simulink model "untitled"  (R2023b)
settings: Solver=VariableStepAuto  StartTime=0.0  StopTime=10.0  RelTol=1e-3
settings Model: Creator=ray  LastModifiedBy=ray

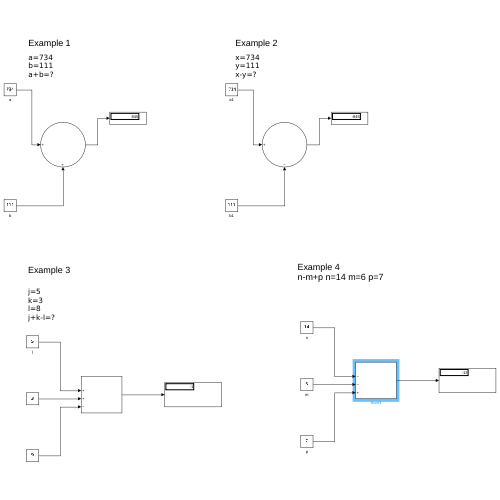
[thumbnail: Simulink's stored preview of the top-level diagram]
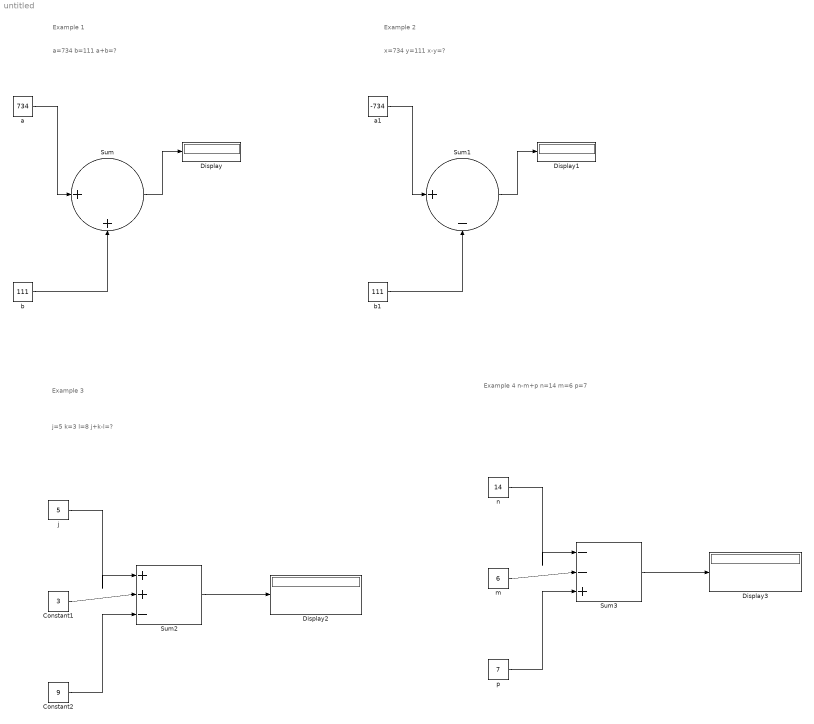
== system untitled ==
  note: a=734
      | b=111
      | a+b=?
  note: Example 1
  note: x=734
      | y=111
      | x-y=?
  note: Example 2
  note: Example 3
  note: j=5
      | k=3
      | l=8
      | j+k-l=?
  note: Example 4
      | n-m+p n=14 m=6 p=7
  Constant1 : Constant  Value=3
  Constant2 : Constant  Value=9
  Display{,1..3} (4 alike) : Display
  Sum : Sum  Inputs=|++
  Sum1 : Sum  Inputs=|+-
  Sum2 : Sum  Inputs=|++-
  Sum3 : Sum  Inputs=|--+
  a : Constant  Value=734
  a1 : Constant  Value=-734
  b : Constant  Value=111
  b1 : Constant  Value=111
  j : Constant  Value=5
  m : Constant  Value=6
  n : Constant  Value=14
  p : Constant  Value=7
  wires:
  a/1 -> Sum/1
  b/1 -> Sum/2
  Sum/1 -> Display/1
  a1/1 -> Sum1/1
  Sum1/1 -> Display1/1
  b1/1 -> Sum1/2
  j/1 -> Sum2/1
  Constant1/1 -> Sum2/2
  Constant2/1 -> Sum2/3
  Sum2/1 -> Display2/1
  p/1 -> Sum3/3
  n/1 -> Sum3/1
  Sum3/1 -> Display3/1
  m/1 -> Sum3/2
